simulink model "three_phase_rectifier_simulation"  (R2023a)
settings: Solver=FixedStepAuto  StartTime=0.0  StopTime=simtime  FixedStep=0.00001  RelTol=1e-3
values from neighbouring files (symbols this model uses):
  C1 = 1.1281e-3    (= 0.0011281)    [three_phase_rectifier_script.m]
  number_of_harmonics = 30    [three_phase_rectifier_script.m]
  R1 = 25    [three_phase_rectifier_script.m]
  simtime = 0.1    [three_phase_rectifier_script.m]
libraries: fl_lib x13, eeGeneralControl x5, nesl_utility x4, spsRMSLib x3, ee_lib x3, simulink x2
settings Model: Creator=citcea  LastModifiedBy=citcea

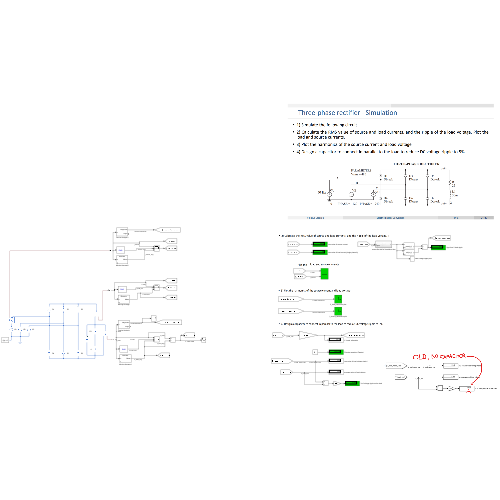
[thumbnail: Simulink's stored preview of the top-level diagram]
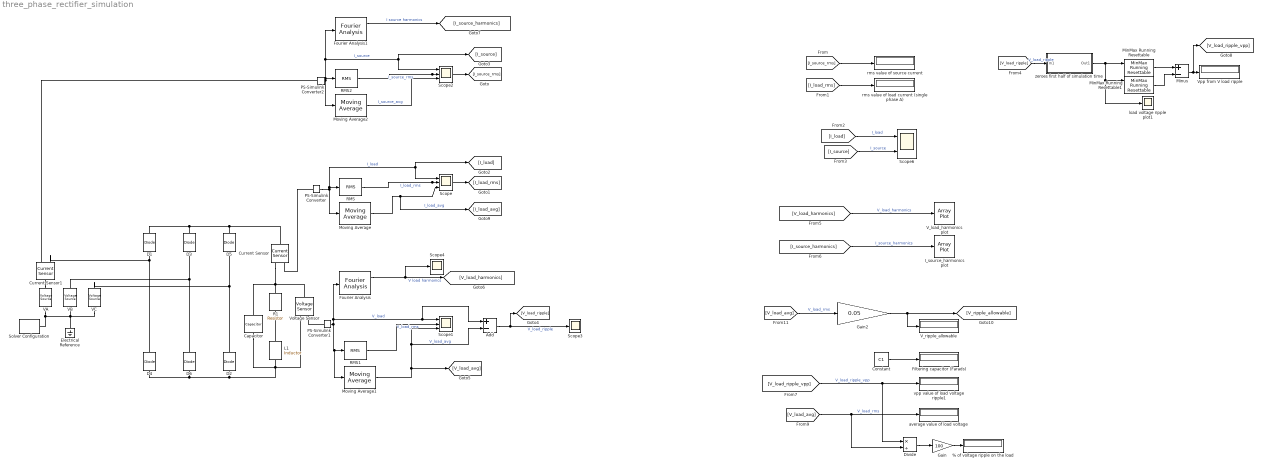
== system three_phase_rectifier_simulation ==
  % of voltage ripple on the load : Display
  Add : Sum  Inputs=+-
  Capacitor : fl_lib/Electrical/Electrical Elements/Capacitor  c=C1 F  r=1e-6 Ohm  g=0 1/Ohm  i_specify=off  i_priority=None  i=0 A  i_nominal_specify=off  i_nominal_unit=A  i_nominal_value=1  v_specify=off  v_priority=None  v=0 V  v_nominal_specify=off  v_nominal_unit=V  v_nominal_value=1  vc_specify=off  vc_priority=High  vc=0 V  vc_nominal_specify=off  vc_nominal_unit=V  vc_nominal_value=1
  Constant : Constant  Value=C1
  Current Sensor : fl_lib/Electrical/Electrical Sensors/Current Sensor
  Current Sensor1 : fl_lib/Electrical/Electrical Sensors/Current Sensor
  D{1..6} (6 alike) : fl_lib/Electrical/Electrical Elements/Diode  Vf=0.6 V  Ron=0.3 Ohm  Goff=1e-8 1/Ohm  i_specify=off  i_priority=None  i=0 A  i_nominal_specify=off  i_nominal_unit=A  i_nominal_value=1  v_specify=off  v_priority=None  v=0 V  v_nominal_specify=off  v_nominal_unit=V  v_nominal_value=1
  Divide : Product  Inputs=*/
  Electrical Reference : fl_lib/Electrical/Electrical Elements/Electrical Reference
  Filtering capacitor (Farads) : Display
  Fourier Analysis : eeGeneralControl/Fourier Analysis  f=source_freq  n=[0:1:number_of_harmonics]  M0=1  Ph0=0  BufferSize=8192  Ts=-1
      settings: LibrarySourceBlock=ee_sl_lib/General Control/Fourier Analysis
  Fourier Analysis1 : eeGeneralControl/Fourier Analysis  f=source_freq  n=[0:1:number_of_harmonics]  M0=1  Ph0=0  BufferSize=8192  Ts=-1
      settings: LibrarySourceBlock=ee_sl_lib/General Control/Fourier Analysis
  Gain : Gain  Gain=100
  Gain2 : Gain  Gain=0.05
  I_source_harmonics plot : ArrayPlot  WindowPosition=[95.000000,148.000000,800.000000,500.000000,]  Visible=on  ScopeFrameLocation=window  YLimits=[-6.3149,56.8338]
  L1 : fl_lib/Electrical/Electrical Elements/Inductor  l=L1 H  r=0 Ohm  g=1e-9 1/Ohm  i_specify=off  i_priority=None  i=0 A  i_nominal_specify=off  i_nominal_unit=A  i_nominal_value=1  v_specify=off  v_priority=None  v=0 V  v_nominal_specify=off  v_nominal_unit=V  v_nominal_value=1  i_L_specify=off  i_L_priority=High  i_L=0 A  i_L_nominal_specify=off  i_L_nominal_unit=A  i_L_nominal_value=1
  MinMax Running Resettable : simulink/Math Operations/MinMax Running Resettable  Function=max  vinit=0.0
  MinMax Running Resettable1 : simulink/Math Operations/MinMax Running Resettable  Function=min  vinit=0.0
  Minus : Sum  Inputs=+-
  Moving Average : eeGeneralControl/Moving Average  VariantControl=Variant1  LabelModeActiveChoice=Discrete  f=source_freq  x0=0  BufferSize=8192  Ts=-1
      settings: LibrarySourceBlock=ee_sl_lib/General Control/Moving Average
  Moving Average1 : eeGeneralControl/Moving Average  VariantControl=Variant1  LabelModeActiveChoice=Discrete  f=source_freq  x0=0  BufferSize=8192  Ts=-1
      settings: LibrarySourceBlock=ee_sl_lib/General Control/Moving Average
  Moving Average2 : eeGeneralControl/Moving Average  VariantControl=Variant1  LabelModeActiveChoice=Discrete  f=source_freq  x0=0  BufferSize=8192  Ts=-1
      settings: LibrarySourceBlock=ee_sl_lib/General Control/Moving Average
  PS-Simulink Converter : nesl_utility/PS-Simulink Converter  PhysicalDomain=network_engine_domain  SubClassName=ps_output  LeftPortType=input  RightPortType=output  PseudoPeriodic=off  Frequencies=[]  VectorFormat=inherit  Unit=inherit  AffineConversion=off
  PS-Simulink Converter1 : nesl_utility/PS-Simulink Converter  PhysicalDomain=network_engine_domain  SubClassName=ps_output  LeftPortType=input  RightPortType=output  PseudoPeriodic=off  Frequencies=[]  VectorFormat=inherit  Unit=inherit  AffineConversion=off
  PS-Simulink Converter2 : nesl_utility/PS-Simulink Converter  PhysicalDomain=network_engine_domain  SubClassName=ps_output  LeftPortType=input  RightPortType=output  PseudoPeriodic=off  Frequencies=[]  VectorFormat=inherit  Unit=inherit  AffineConversion=off
  R1 : fl_lib/Electrical/Electrical Elements/Resistor  R=R1 Ohm  i_specify=off  i_priority=None  i=0 A  i_nominal_specify=off  i_nominal_unit=A  i_nominal_value=1  v_specify=off  v_priority=None  v=0 V  v_nominal_specify=off  v_nominal_unit=V  v_nominal_value=1
  RMS : spsRMSLib/RMS  TrueRMS=on  Freq=source_freq  RMSInit=0  Ts=0
  RMS1 : spsRMSLib/RMS  TrueRMS=on  Freq=source_freq  RMSInit=0  Ts=0
  RMS2 : spsRMSLib/RMS  TrueRMS=on  Freq=source_freq  RMSInit=0  Ts=0
  Scope : Scope  NumInputPorts=3
  Scope1 : Scope  NumInputPorts=3
  Scope2 : Scope  NumInputPorts=3
  Scope3 : Scope
  Scope4 : Scope
  Scope6 : Scope  NumInputPorts=2
  Solver Configuration : nesl_utility/Solver Configuration  PhysicalDomain=network_engine_domain  SubClassName=solver  LeftPortType=input  RightPortType=generic  Tones=[]  Harmonics=[]  SimulateNoise=off  Profile=off  UseLocalSampling=off  EnableSwitchedLinearOptims=on  FrequencyDomain=off  UseCCode=off  RelTol=0.001  AbsTol=0.001  MinStep=1e-09  ToWorkspace=off  RevertToSquareIcSolve=off  NumHomotopyIterations=100  PhasorMode=off  PhasorModeNumHarmonics=1  ConsistencySolver=NEWTON_XTOL_AFTER_FTOL  IndexReductionMethod=DerivativeReplacement  DoDC=off  ResidualTolerance=1e-09  ConsistencyTolSource=GLOBAL  ConsistencyAbsTol=0.001  ConsistencyRelTol=0.001  ConsistencyTolFactor=0.001  UseLocalSolver=on  LocalSolverChoice=NE_TRAPEZOIDAL_ADVANCER  ResolveIndetEquations=on  FunctionEvalNumThread=1  LocalSolverSampleTime=50e-6  DoFixedCost=on  MaxNonlinIter=3  MaxModeIter=2  ComputeImpulses=off  ImpulseIterations=2  LinearAlgebra=auto  LinearAlgebraNumThread=0  EquationFormulation=NE_TIME_EF  DelaysMemoryBudget=1024  AutomaticFiltering=on  FilteringTimeConstant=0.001  PartitionStorageMethod=AS_NEEDED  PartitionMemoryBudget=1024  PartitionMethod=ROBUST
  VA : ee_lib/Sources/Voltage Source  dc_voltage=0 V  ac_voltage=Vpeak V  ac_shift=source_phase_shiftA deg  ac_frequency=source_freq Hz  noise_mode=ee.enum.sources.noise.Disabled  PSD=0 V^2/Hz  sample_time=1e-3 s  repeatability=ee.enum.sources.repeatability.NotRepeatable  user_seed=0  auto_seed=3499211588  i_specify=off  i_priority=None  i=0 A  i_nominal_specify=off  i_nominal_unit=A  i_nominal_value=1  v_specify=off  v_priority=None  v=0 V  v_nominal_specify=off  v_nominal_unit=V  v_nominal_value=1
  "VB " : ee_lib/Sources/Voltage Source  dc_voltage=0 V  ac_voltage=Vpeak V  ac_shift=source_phase_shiftB deg  ac_frequency=source_freq Hz  noise_mode=ee.enum.sources.noise.Disabled  PSD=0 V^2/Hz  sample_time=1e-3 s  repeatability=ee.enum.sources.repeatability.NotRepeatable  user_seed=0  auto_seed=3890346746  i_specify=off  i_priority=None  i=0 A  i_nominal_specify=off  i_nominal_unit=A  i_nominal_value=1  v_specify=off  v_priority=None  v=0 V  v_nominal_specify=off  v_nominal_unit=V  v_nominal_value=1
  VC : ee_lib/Sources/Voltage Source  dc_voltage=0 V  ac_voltage=Vpeak V  ac_shift=source_phase_shiftC deg  ac_frequency=source_freq Hz  noise_mode=ee.enum.sources.noise.Disabled  PSD=0 V^2/Hz  sample_time=1e-3 s  repeatability=ee.enum.sources.repeatability.NotRepeatable  user_seed=0  auto_seed=545404223  i_specify=off  i_priority=None  i=0 A  i_nominal_specify=off  i_nominal_unit=A  i_nominal_value=1  v_specify=off  v_priority=None  v=0 V  v_nominal_specify=off  v_nominal_unit=V  v_nominal_value=1
  V_load_harmonics plot : ArrayPlot  WindowPosition=[1.000000,49.000000,1536.000000,889.000000,]  ScopeFrameLocation=window  YLimits=[-138.3757,1245.3812]
  V_ripple_allowable : Display
  Voltage Sensor : fl_lib/Electrical/Electrical Sensors/Voltage Sensor
  Vpp from V load ripple : Display
  average value of load voltage : Display
  load voltage ripple plot1 : Scope
  rms value of load current (single phase A) : Display
  rms value of source current : Display
  vpp value of load voltage ripple1 : Display
  zeroes first half of simulation time : Subsystem
  wires:
  PS-Simulink Converter/1 -> [I_load], Scope/1, RMS/1, Moving Average/1  "I_load"
  RMS/1 -> [I_load_rms], Scope/2  "I_load_rms"
  Moving Average/1 -> [I_load_avg], Scope/3  "I_load_avg"
  RMS1/1 -> Scope1/2  "V_load_rms"
  Moving Average1/1 -> [V_load_avg], Scope1/3, Add/2  "V_load_avg"
  Moving Average2/1 -> Scope2/3  "I_source_avg"
  PS-Simulink Converter2/1 -> Fourier Analysis1/1, [I_source], Scope2/1, RMS2/1, Moving Average2/1  "I_source"
  RMS2/1 -> [I_source_rms], Scope2/2  "I_source_rms"
  Add/1 -> [V_load_ripple], Scope3/1  "V_load_ripple"
  PS-Simulink Converter1/1 -> Moving Average1/1, RMS1/1, Fourier Analysis/1, Add/1, Scope1/1  "V_load"
  Fourier Analysis/1 -> Scope4/1, [V_load_harmonics]  "V load harmonics"
  Fourier Analysis1/1 -> [I_source_harmonics]  "I source harmonics"
  [I_source_rms] -> rms value of source current/1
  [I_load_rms] -> rms value of load current (single phase A)/1
  [I_load] -> Scope6/1  "I_load"
  [I_source] -> Scope6/2  "I_source"
  [V_load_ripple] -> zeroes first half of simulation time/1(In1)  "V_load_ripple"
  [V_load_harmonics] -> V_load_harmonics plot/1  "V_load_harmonics"
  [I_source_harmonics] -> I_source_harmonics plot/1  "I_source_harmonics"
  [V_load_ripple_vpp] -> Divide/1, vpp value of load voltage ripple1/1  "V_load_ripple_vpp"
  [V_load_avg] -> average value of load voltage/1, Divide/2  "V_load_rms"
  Divide/1 -> Gain/1
  Gain/1 -> % of voltage ripple on the load/1
  MinMax Running Resettable1/1 -> Minus/2
  zeroes first half of simulation time/1(Out1) -> load voltage ripple plot1/1, MinMax Running Resettable1/1, MinMax Running Resettable/1
  MinMax Running Resettable/1 -> Minus/1
  Minus/1 -> [V_load_ripple_vpp], Vpp from V load ripple/1
  Gain2/1 -> V_ripple_allowable/1, [V_ripple_allowable]
  [V_load_avg] -> Gain2/1  "V_load_rms"
  Constant/1 -> Filtering capacitor (Farads)/1
  connections:
  "VB "/RConn1 -- Solver Configuration/RConn1 -- VA/RConn1 -- Electrical Reference/LConn1 -- VC/RConn1
  D4/RConn1 -- Current Sensor1/RConn2 -- D1/LConn1
  "VB "/LConn1 -- D3/LConn1 -- D6/RConn1
  VC/LConn1 -- D2/RConn1 -- D5/LConn1
  D2/LConn1 -- Capacitor/RConn1 -- Voltage Sensor/RConn2 -- L1/RConn1 -- D4/LConn1 -- D6/LConn1
  D1/RConn1 -- Current Sensor/LConn1 -- D5/RConn1 -- D3/RConn1
  L1/LConn1 -- R1/RConn1
  Current Sensor/RConn2 -- Capacitor/LConn1 -- Voltage Sensor/LConn1 -- R1/LConn1
  PS-Simulink Converter/LConn1 -- Current Sensor/RConn1
  PS-Simulink Converter1/LConn1 -- Voltage Sensor/RConn1
  Current Sensor1/LConn1 -- VA/LConn1
  PS-Simulink Converter2/LConn1 -- Current Sensor1/RConn1

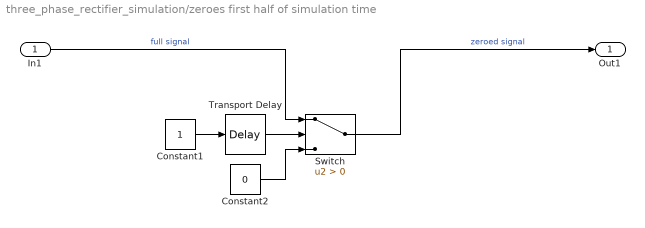
== system three_phase_rectifier_simulation/zeroes first half of simulation time ==
  In1 : Inport
  Constant1 : Constant
  Constant2 : Constant  Value=0
  Switch : Switch  Criteria=u2 > Threshold  SaturateOnIntegerOverflow=off  InputSameDT=off
  Transport Delay : TransportDelay  DelayTime=simtime/2
  Out1 : Outport
  wires:
  Constant1/1 -> Transport Delay/1
  Constant2/1 -> Switch/3
  Transport Delay/1 -> Switch/2
  In1/1 -> Switch/1  "full signal"
  Switch/1 -> Out1/1  "zeroed signal"
